simulink model "i_controller"  (R2022a)
settings: Solver=VariableStepAuto  StartTime=0.0  StopTime=10.0  RelTol=1e-3
settings Model: Creator=Laptop-Academy.com  LastModifiedBy=Laptop-Academy.com

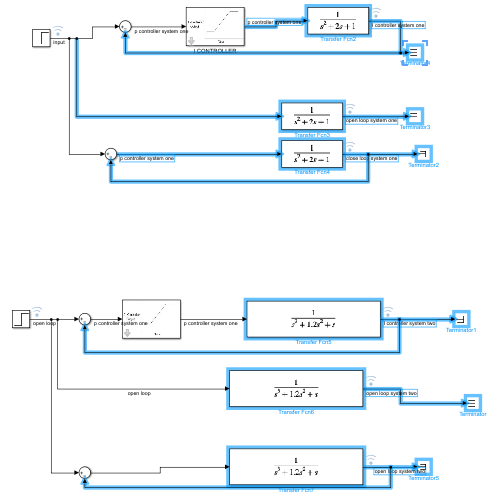
[thumbnail: Simulink's stored preview of the top-level diagram]
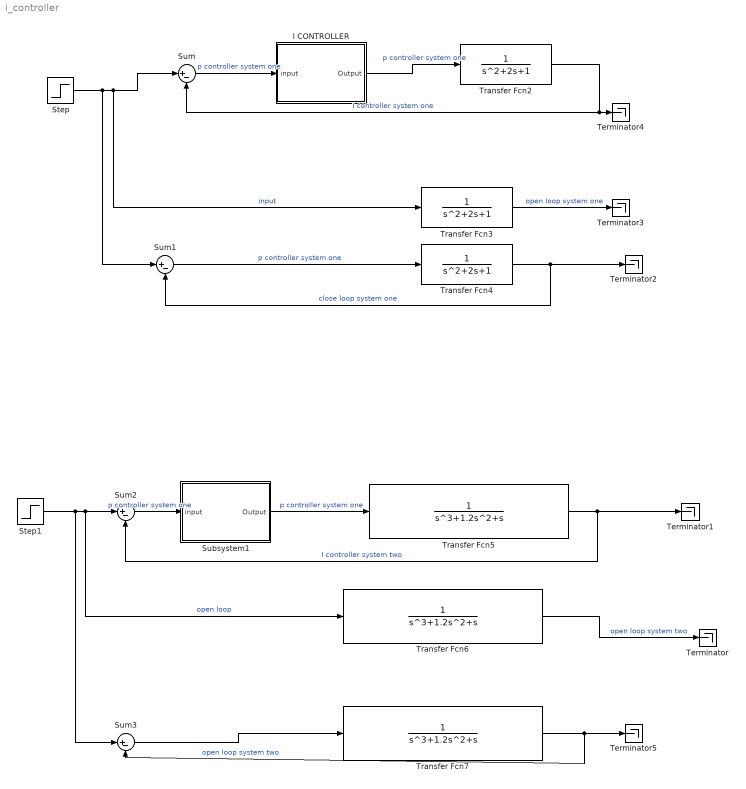
== system i_controller ==
  I CONTROLLER : Subsystem  mask{i=0}
      mask prompts: i "integrator gain (I)"
      mask DialogControl DescGroupVar Prompt: integral controller
      mask DialogControl DescTextVar Prompt: this is integral controller
      mask Display: image("F:\os_academy_labs\pid_controller\media\i.jpg");
  Step : Step  SampleTime=0
  Step1 : Step  SampleTime=0
  Subsystem1 : Subsystem  mask{i=0}
      mask prompts: i "integrator gain (I)"
      mask DialogControl DescGroupVar Prompt: integral controller
      mask DialogControl DescTextVar Prompt: this is integral controller
      mask Display: image("F:\os_academy_labs\pid_controller\media\i.jpg");
  Sum{,1..3} (4 alike) : Sum  Inputs=|+-
  Terminator{,1..5} (6 alike) : Terminator
  Transfer Fcn2 : TransferFcn
  Transfer Fcn3 : TransferFcn
  Transfer Fcn4 : TransferFcn
  Transfer Fcn5 : TransferFcn  Denominator=[1 1.2 1 0]
  Transfer Fcn6 : TransferFcn  Denominator=[1 1.2 1 0]
  Transfer Fcn7 : TransferFcn  Denominator=[1 1.2 1 0]
  wires:
  Step1/1 -> Sum3/1, Transfer Fcn6/1, Sum2/1  "open loop"
  Transfer Fcn5/1 -> Sum2/2, Terminator1/1  "I controller system two"
  I CONTROLLER/1(Output) -> Transfer Fcn2/1  "p controller system one"
  Transfer Fcn7/1 -> Sum3/2, Terminator5/1  "open loop system two"
  Transfer Fcn6/1 -> Terminator/1  "open loop system two"
  Transfer Fcn3/1 -> Terminator3/1  "open loop system one"
  Transfer Fcn2/1 -> Sum/2, Terminator4/1  "I controller system one"
  Transfer Fcn4/1 -> Sum1/2, Terminator2/1  "close loop system one"
  Sum3/1 -> Transfer Fcn7/1
  Sum/1 -> I CONTROLLER/1(input)  "p controller system one"
  Step/1 -> Sum1/1, Transfer Fcn3/1, Sum/1  "input"
  Sum1/1 -> Transfer Fcn4/1  "p controller system one"
  Subsystem1/1(Output) -> Transfer Fcn5/1  "p controller system one"
  Sum2/1 -> Subsystem1/1(input)  "p controller system one"

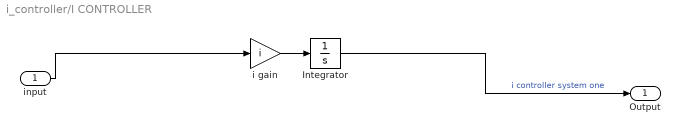
== system i_controller/I CONTROLLER ==
  input : Inport
  Integrator : Integrator
  i gain : Gain  Gain=i
  Output : Outport
  wires:
  input/1 -> i gain/1
  i gain/1 -> Integrator/1
  Integrator/1 -> Output/1  "i controller system one"

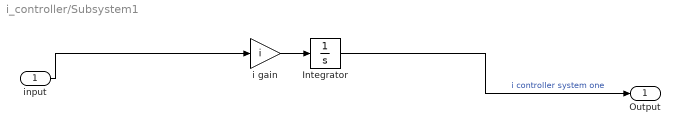
== system i_controller/Subsystem1 ==
  input : Inport
  Integrator : Integrator
  i gain : Gain  Gain=i
  Output : Outport
  wires:
  Integrator/1 -> Output/1  "i controller system one"
  i gain/1 -> Integrator/1
  input/1 -> i gain/1
